simulink model "lqg_cartpend_sim"  (R2019a)
settings: Solver=VariableStepAuto  StartTime=0.0  StopTime=50.0  RelTol=1e-3  EnableMultiTasking=on
values from neighbouring files (symbols this model uses):
  C = [1 0 0 0]    [lqg_simulinkINIT.m]
  K = lqr(A,B,Q,R)    [lqg_simulinkINIT.m]
  sysKF = ss(A_estimation-Kf*C1,[B_estimation Kf],eye(4),0*[B_estimation Kf])    [inverted_pendulum_control.m]    (also in lqg_simulinkINIT.m = ss(A-Kf*C,[B Kf],eye(4),0*[B Kf]))
settings Model: Creator=sbrunton  LastModifiedBy=Aalap
settings DataIOCC: LimitDataPoints=on  ReturnWorkspaceOutputs=off
settings OptimizationCC: LifeSpan=inf
settings DebuggingCC: AllowSymbolicDim=off  SFUnexpectedBacktrackingDiag=warning  SFNoUnconditionalDefaultTransitionDiag=warning  SFExecutionAtInitializationDiag=none  ArithmeticOperatorsInVariantConditions=warning
settings ModelReferenceCC: PropagateSignalLabelsOutOfModel=off
settings SFSimCC: SimUseLocalCustomCode=off
settings RTWCC: RTWUseLocalCustomCode=off
settings CodeAppCC: StateflowObjectComments=on
settings GRTTargetCC: TargetLangStandard=C89/C90 (ANSI)
settings ConfigComp: CovMetricSettings=dw  CovHtmlReporting=on  CovSaveCumulativeToWorkspaceVar=on  CovSaveSingleToWorkspaceVar=on  CovExternalEMLEnable=off

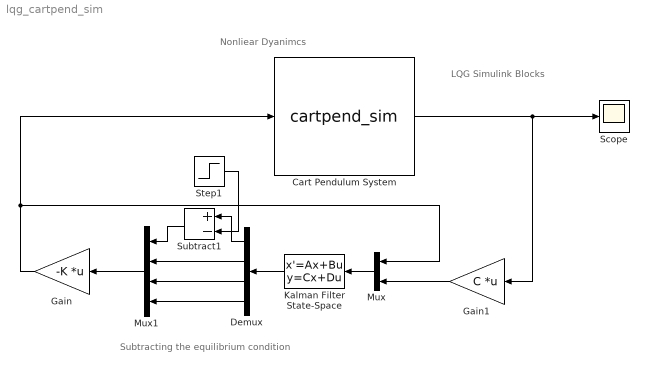
== system lqg_cartpend_sim ==
  note: Subtracting the equilibrium condition
  note: Nonliear Dyanimcs
  note: LQG Simulink Blocks
  " Kalman Filter State-Space" : StateSpace  A=sysKF.a  B=sysKF.b  C=sysKF.c  D=sysKF.d  InitialCondition=[0 0 0 0]
  "Cart Pendulum System " : S-Function  InitFcn=try, set_param(gcb,'FunctionName','cartpend_sim'), end  FunctionName=cartpend_sim  SFunctionModules=cartpend_sim_wrapper  SFunctionDeploymentMode=off  EnableBusSupport=off  mask(S-Function Builder){}
      mask help: Simulink:masks:SFunctionBuilder_MD
      mask init:
      | val = [[.9  0.75 0.75 1 1 .9 .9 1]',[1 1 0.75 0.75 .9 .9 1 .9]'];try , sys = get_param(gcb,'SfunBuilderFcnName');if isempty(sys), sys = get_param(gcb,'FunctionName'); end,catch, sys = get_param(gcb,'FunctionName'); end
      settings: CopyFcn=set_param(gcbh,'LinkStatus','none')  PreSaveFcn=try, set_param(gcb,'FunctionName','cartpend_sim'), end  OpenFcn=sfunctionwizard(gcbh)
      mask Display: plot(val(:,1),val(:,2)),disp(sys), port_label('input',1,'u0'), port_label('output',1,'y0')
  Demux : Demux
  Gain : Gain  Gain=-K  Multiplication=Matrix(K*u) (u vector)
  Gain1 : Gain  Gain=C  Multiplication=Matrix(K*u) (u vector)
  Mux : Mux  Inputs=2
  Mux1 : Mux
  Scope : Scope
  Step1 : Step  Time=10  SampleTime=0
  Subtract1 : Sum  Inputs=+-
  wires:
  Gain/1 -> Mux/1, "Cart Pendulum System "/1
  "Cart Pendulum System "/1 -> Gain1/1, Scope/1
  Mux/1 -> " Kalman Filter State-Space"/1
  Demux/2 -> Mux1/2
  Demux/4 -> Mux1/4
  Demux/3 -> Mux1/3
  Mux1/1 -> Gain/1
  Subtract1/1 -> Mux1/1
  Demux/1 -> Subtract1/1
  Step1/1 -> Subtract1/2
  " Kalman Filter State-Space"/1 -> Demux/1
  Gain1/1 -> Mux/2
